simulink library "sun_point_lib"  (R2016b)
settings: Solver=VariableStepAuto  StartTime=0.0  StopTime=10.0  RelTol=1e-3
undefined symbols (not defined in the file or in its folder): fsw_params
libraries: vrlib x1, dspmathops x1
settings Model: Creator=Krish  LastModifiedBy=Krish

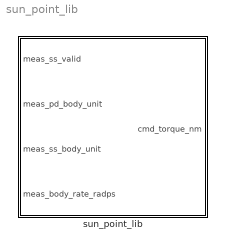
== system sun_point_lib ==
  sun_point_lib : Subsystem  TreatAsAtomicUnit=on
      settings: MinAlgLoopOccurrences=on  RTWFcnNameOpts=Use subsystem name  RTWFileNameOpts=Use subsystem name

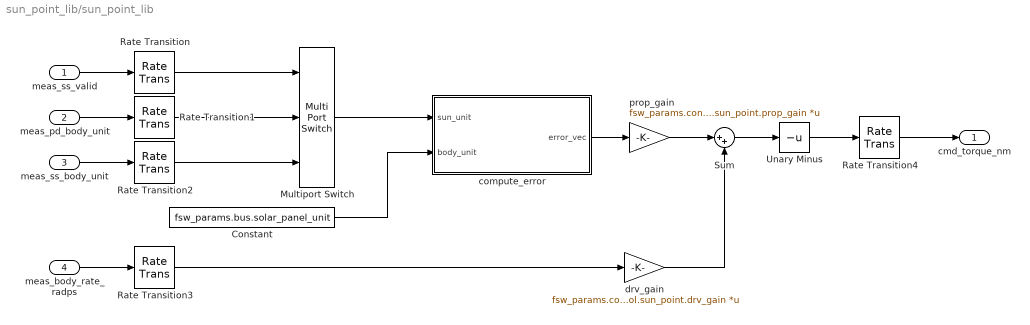
== system sun_point_lib/sun_point_lib ==
  meas_ss_valid : Inport
  meas_pd_body_unit : Inport  Port=2
  meas_ss_body_unit : Inport  Port=3
  meas_body_rate_radps : Inport  Port=4
  Constant : Constant  Value=fsw_params.bus.solar_panel_unit
  Multiport Switch : MultiPortSwitch  DataPortOrder=Zero-based contiguous  Inputs=2
  Rate Transition : RateTransition  X0=fsw_params.control.sun_point.ic.meas_ss_valid  OutPortSampleTime=fsw_params.control.sun_point.sample_time_s
  Rate Transition1 : RateTransition  X0=fsw_params.control.sun_point.ic.meas_pd_body_unit  OutPortSampleTime=fsw_params.control.sun_point.sample_time_s
  Rate Transition2 : RateTransition  X0=fsw_params.control.sun_point.ic.meas_ss_body_unit  OutPortSampleTime=fsw_params.control.sun_point.sample_time_s
  Rate Transition3 : RateTransition  X0=fsw_params.control.sun_point.ic.meas_body_rate_radps  OutPortSampleTime=fsw_params.control.sun_point.sample_time_s
  Rate Transition4 : RateTransition  X0=fsw_params.control.sun_point.ic.cmd_torque_nm  OutPortSampleTimeOpt=Inherit
  Sum : Sum  Inputs=|++
  Unary Minus : UnaryMinus
  compute_error : Subsystem
  drv_gain : Gain  Gain=fsw_params.control.sun_point.drv_gain  Multiplication=Matrix(K*u)
  prop_gain : Gain  Gain=fsw_params.control.sun_point.prop_gain  Multiplication=Matrix(K*u)
  cmd_torque_nm : Outport
  wires:
  Multiport Switch/1 -> compute_error/1(sun_unit)
  Rate Transition/1 -> Multiport Switch/1
  Rate Transition1/1 -> Multiport Switch/2
  Rate Transition3/1 -> drv_gain/1
  meas_pd_body_unit/1 -> Rate Transition1/1
  compute_error/1(error_vec) -> prop_gain/1
  meas_ss_valid/1 -> Rate Transition/1
  Rate Transition2/1 -> Multiport Switch/3
  drv_gain/1 -> Sum/2
  Constant/1 -> compute_error/2(body_unit)
  meas_ss_body_unit/1 -> Rate Transition2/1
  prop_gain/1 -> Sum/1
  meas_body_rate_radps/1 -> Rate Transition3/1
  Sum/1 -> Unary Minus/1
  Unary Minus/1 -> Rate Transition4/1
  Rate Transition4/1 -> cmd_torque_nm/1

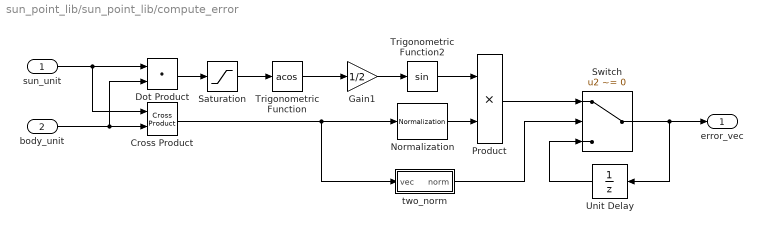
== system sun_point_lib/sun_point_lib/compute_error ==
  sun_unit : Inport
  body_unit : Inport  Port=2
  Cross Product : vrlib/Utilities/Cross Product
  Dot Product : DotProduct  InputSameDT=on  OutDataTypeStr=Inherit: Inherit via internal rule
  Gain1 : Gain  Gain=1/2
  Normalization : dspmathops/Normalization  NormType=2-norm  Bias=1e-10  NormOver=Each column  Dimension=1  outputDataTypeStr=Inherit: Same as product output  outputLastDataTypeStr=Inherit: Same as product output  outputMin=[]  outputMax=[]  accumDataTypeStr=Inherit: Same as product output  accumLastDataTypeStr=Inherit: Same as product output  roundingMode=Floor  overflowMode=off
  Product : Product
  Saturation : Saturate  UpperLimit=1  LowerLimit=-1
  Switch : Switch  Criteria=u2 ~= 0
  Trigonometric Function : Trigonometry  Operator=acos
  Trigonometric Function2 : Trigonometry
  Unit Delay : UnitDelay  InitialCondition=fsw_params.control.sun_point.ic.error_vec  SampleTime=-1
  two_norm : Subsystem
  error_vec : Outport
  wires:
  body_unit/1 -> Dot Product/2, Cross Product/2
  Trigonometric Function2/1 -> Product/1
  Product/1 -> Switch/1
  sun_unit/1 -> Cross Product/1, Dot Product/1
  Saturation/1 -> Trigonometric Function/1
  Gain1/1 -> Trigonometric Function2/1
  Normalization/1 -> Product/2
  Trigonometric Function/1 -> Gain1/1
  Dot Product/1 -> Saturation/1
  Cross Product/1 -> Normalization/1, two_norm/1(vec)
  Switch/1 -> Unit Delay/1, error_vec/1
  Unit Delay/1 -> Switch/3
  two_norm/1(norm) -> Switch/2

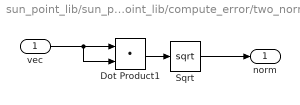
== system sun_point_lib/sun_point_lib/compute_error/two_norm ==
  vec : Inport
  Dot Product1 : DotProduct  InputSameDT=on  OutDataTypeStr=Inherit: Inherit via internal rule
  Sqrt : Sqrt  SaturateOnIntegerOverflow=on
  norm : Outport
  wires:
  vec/1 -> Dot Product1/2, Dot Product1/1
  Dot Product1/1 -> Sqrt/1
  Sqrt/1 -> norm/1
